simulink model "myexp5_2"  (R2022a)
settings: Solver=VariableStepAuto  StartTime=0.0  StopTime=100000  RelTol=1e-3
values from neighbouring files (symbols this model uses):
  n = n_list(i)    [exp5.m]    (also in exp5h.m = 2^M - 1)
libraries: commrandsrc3 x1, commchan3 x1, commsink2 x1
settings Model: Creator=惠普  LastModifiedBy=惠普

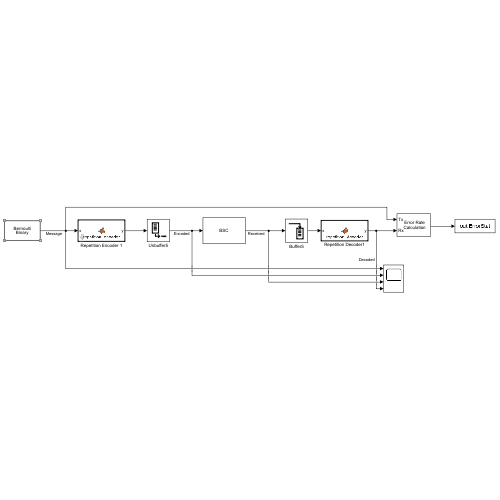
[thumbnail: Simulink's stored preview of the top-level diagram]
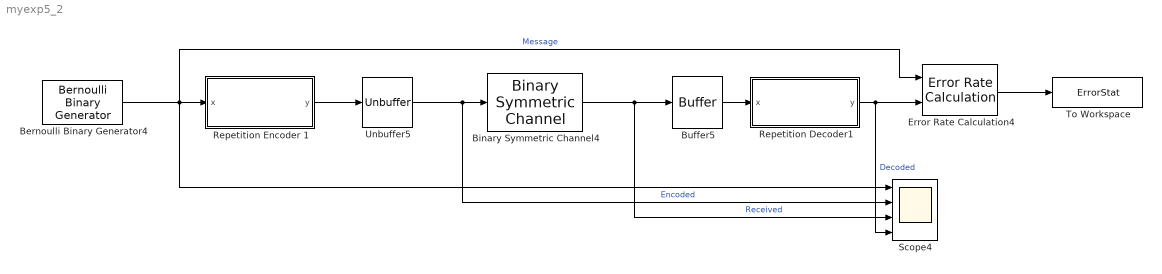
== system myexp5_2 ==
  Bernoulli Binary Generator4 : commrandsrc3/Bernoulli Binary Generator  ProbabilityOfZero=0.5  SeedSource=Auto  Seed=0  SampleTime=1  SamplesPerFrame=1  OutputDataType=double  SimulateUsing=Interpreted execution
  Binary Symmetric Channel4 : commchan3/Binary Symmetric Channel  ErrorProbability=eprob  ErrorVectorOutputPort=off  OutputDataType=double  OutputDataTypeSL=double  Seed=137  SimulateUsing=Code generation
      settings: SourceProductBaseCode=CM
  Buffer5 : Buffer  N=n  OutputFrames=off
  Error Rate Calculation4 : commsink2/Error Rate Calculation  N=1  st_delay=0  cp_mode=Entire frame  subframe=[]  PMode=Port  WsName=ErrorVec  RsMode2=off  stop=off  numErr=100  maxBits=1e6
  Repetition Decoder1 : MATLAB Function  TreatAsAtomicUnit=on
  Repetition Encoder 1 : MATLAB Function  TreatAsAtomicUnit=on  mask{n=n}
      mask prompts: n "number of repetitions"
  Scope4 : Scope  NumInputPorts=4
  To Workspace : ToWorkspace  VariableName=ErrorStat  SampleTime=-1
      settings: MaxDataPoints=1
  Unbuffer5 : Unbuffer
  wires:
  Repetition Encoder 1/1(y) -> Unbuffer5/1
  Binary Symmetric Channel4/1 -> Scope4/3, Buffer5/1  "Received"
  Error Rate Calculation4/1 -> To Workspace/1
  Unbuffer5/1 -> Scope4/2, Binary Symmetric Channel4/1  "Encoded"
  Repetition Decoder1/1(y) -> Scope4/4, Error Rate Calculation4/2  "Decoded"
  Bernoulli Binary Generator4/1 -> Error Rate Calculation4/1, Scope4/1, Repetition Encoder 1/1(x)  "Message"
  Buffer5/1 -> Repetition Decoder1/1(x)

== matlab function myexp5_2/Repetition Encoder 1 ==
  data: x input; y output; n parameter
function y = repetition_encoder(x, n)
y = repelem([x],n)';

== matlab function myexp5_2/Repetition Decoder1 ==
  data: x input; y output
function y = repetition_decoder(x)
n0 = length(find(x == 0));
n1 = length(find(x == 1));
if(n0 >= n1)
    y = 0;
else
    y = 1;
end
